simulink model "dee"  (R2014b)
settings: Solver=ode45  SolverMode=SingleTasking  StartTime=0.0  StopTime=600  RelTol=1e-3  AbsTol=1e-6
values from neighbouring files (symbols this model uses):
  a = 1.0    (= 1)    [DinamicSystemLab6.m]
  alf = -1.6    [DinamicSystemLab6.m]
  b = 3.0    (= 3)    [DinamicSystemLab6.m]
  c = 1.0    (= 1)    [DinamicSystemLab6.m]
  d = 5.0    (= 5)    [DinamicSystemLab6.m]
  I = 2.7    [DinamicSystemLab6.m]    (also in Slony.m = imread('9.jpg'))
  r = 0.003    [DinamicSystemLab6.m]
  s = 4.0    (= 4)    [DinamicSystemLab6.m]
libraries: simulink x1
settings Model: ExtModeTrigMode=oneshot  ExtModeArmWhenConnect=off  Creator=sanjai  LastModifiedBy=student
settings DataIOCC: LimitDataPoints=off  SignalLoggingSaveFormat=ModelDataLogs  SaveOutput=off  SaveTime=off
settings OptimizationCC: BlockReduction=off  BooleanDataType=off
settings DebuggingCC: SaveWithParameterizedLinksMsg=none  UnderspecifiedInitializationDetection=Classic  MergeDetectMultiDrivingBlocksExec=none  SignalResolutionControl=TryResolveAllWithWarning  SolverPrmCheckMsg=none  MultiTaskDSMMsg=warning  MultiTaskCondExecSysMsg=none
settings HardwareCC: TargetUnknown=on
settings RTWCC: IncludeERTFirstTime=on
settings GRTTargetCC: CombineOutputUpdateFcns=off  GRTInterface=on

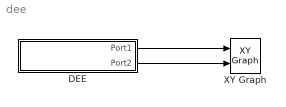
== system dee ==
  DEE : Subsystem  mask(Differential Equation Editor (DEE)){}
      settings: OpenFcn=diffeqed
      mask Display: disp('HindmarshRose\nHR3')
  XY Graph : simulink/Sinks/XY Graph  xmin=-10  xmax=10  ymin=-15  ymax=5  st=-1
  wires:
  DEE/1(Port1) -> XY Graph/1
  DEE/2(Port2) -> XY Graph/2

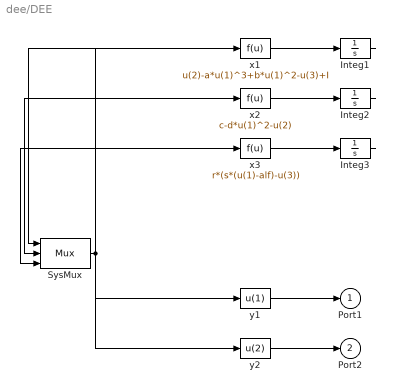
== system dee/DEE ==
  Integ1 : Integrator  InitialCondition=-1
  Integ2 : Integrator
  Integ3 : Integrator  InitialCondition=1
  SysMux : Mux  Inputs=3
  x1 : Fcn  Expr=u(2)-a*u(1)^3+b*u(1)^2-u(3)+I
  x2 : Fcn  Expr=c-d*u(1)^2-u(2)
  x3 : Fcn  Expr=r*(s*(u(1)-alf)-u(3))
  y1 : Fcn  Expr=u(1)
  y2 : Fcn  Expr=u(2)
  Port1 : Outport
  Port2 : Outport  Port=2
  wires:
  SysMux/1 -> x1/1, x2/1, x3/1, y1/1, y2/1
  x1/1 -> Integ1/1
  Integ1/1 -> SysMux/1
  x2/1 -> Integ2/1
  Integ2/1 -> SysMux/2
  x3/1 -> Integ3/1
  Integ3/1 -> SysMux/3
  y1/1 -> Port1/1
  y2/1 -> Port2/1
